simulink subsystem "lat_velocity_generator"  (R2019b)
settings: Solver=VariableStepAuto  StartTime=0.0  StopTime=10.0  RelTol=1e-3
model mask{lat_vel_error_gain=0, deadzone_bound=0, override_time=0}
  mask prompts: lat_vel_error_gain "Proportial Speed Gain"; deadzone_bound "Proportial Speed Deadzone Bound (m/s)"; override_time "Max Velocity Override Time (s)"
undefined symbols (not defined in the file): abs_yaw_params, counter_max, speed
libraries: simulink x2
settings Model: Creator=andrea  LastModifiedBy=andrea

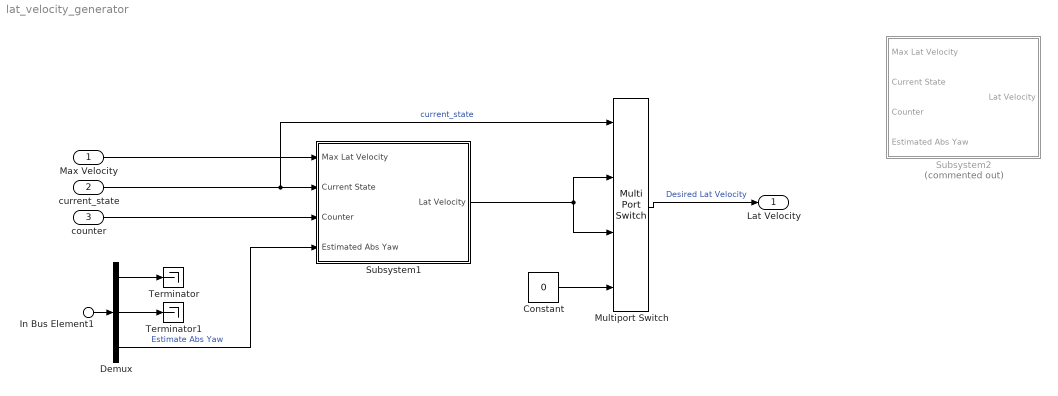
== system lat_velocity_generator ==
  Max Velocity : Inport
  current_state : Inport  Port=2
  counter : Inport  Port=3
  In Bus Element1 : Inport  Port=4  PortName=Estimates Bus  Element=Estimated Abs Orientation
  Constant : Constant  Value=0
  Demux : Demux  Outputs=3
  Multiport Switch : MultiPortSwitch  DataPortOrder=Specify indices  DataPortIndices={103, 202, 201}  DiagnosticForDefault=None
  Subsystem1 : Subsystem
  Subsystem2 : Subsystem  Commented=on
  Terminator : Terminator
  Terminator1 : Terminator
  Lat Velocity : Outport
  wires:
  Max Velocity/1 -> Subsystem1/1(Max Lat Velocity)
  current_state/1 -> Multiport Switch/1, Subsystem1/2(Current State)  "current_state"
  counter/1 -> Subsystem1/3(Counter)
  Demux/3 -> Subsystem1/4(Estimated Abs Yaw)  "Estimate Abs Yaw"
  In Bus Element1/1 -> Demux/1
  Demux/1 -> Terminator/1
  Demux/2 -> Terminator1/1
  Multiport Switch/1 -> Lat Velocity/1  "Desired Lat Velocity"
  Subsystem1/1(Lat Velocity) -> Multiport Switch/3, Multiport Switch/2
  Constant/1 -> Multiport Switch/4

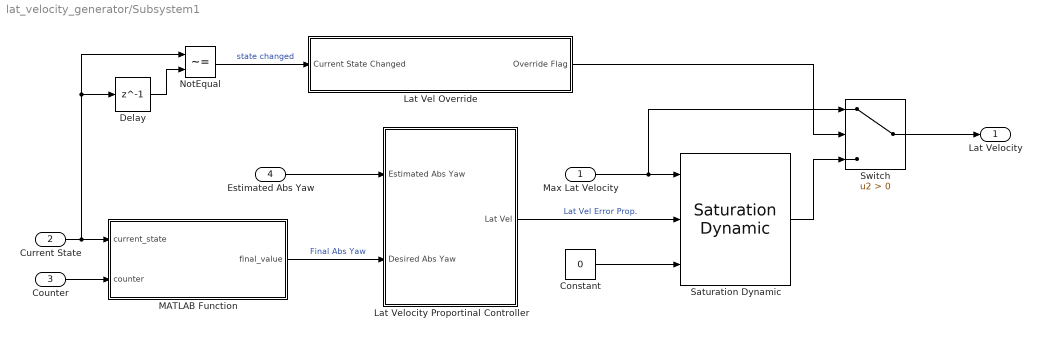
== system lat_velocity_generator/Subsystem1 ==
  Max Lat Velocity : Inport
  Current State : Inport  Port=2
  Counter : Inport  Port=3
  Estimated Abs Yaw : Inport  Port=4
  Constant : Constant  Value=0
  Delay : Delay  DelayLength=1
  Lat Vel Override : Subsystem
  Lat Velocity Proportinal Controller : Subsystem
  MATLAB Function : MATLAB Function  TreatAsAtomicUnit=on
  NotEqual : RelationalOperator  Operator=~=  OutDataTypeStr=boolean  RndMeth=Simplest
  Saturation Dynamic : simulink/Discontinuities/Saturation Dynamic  OutMin=[]  OutMax=[]  OutDataTypeStr=Inherit: Same as second input  OutDataType=fixdt(1, 16)  OutScaling=2^-10  DoSatur=off
  Switch : Switch  Criteria=u2 > Threshold
  Lat Velocity : Outport
  wires:
  Switch/1 -> Lat Velocity/1
  Lat Vel Override/1(Override Flag) -> Switch/2
  NotEqual/1 -> Lat Vel Override/1(Current State Changed)  "state changed"
  Delay/1 -> NotEqual/2
  MATLAB Function/1(final_value) -> Lat Velocity Proportinal Controller/2(Desired Abs Yaw)  "Final Abs Yaw"
  Current State/1 -> MATLAB Function/1(current_state), NotEqual/1, Delay/1
  Max Lat Velocity/1 -> Saturation Dynamic/1, Switch/1
  Saturation Dynamic/1 -> Switch/3
  Constant/1 -> Saturation Dynamic/3
  Counter/1 -> MATLAB Function/2(counter)
  Estimated Abs Yaw/1 -> Lat Velocity Proportinal Controller/1(Estimated Abs Yaw)
  Lat Velocity Proportinal Controller/1(Lat Vel) -> Saturation Dynamic/2  "Lat Vel Error Prop."

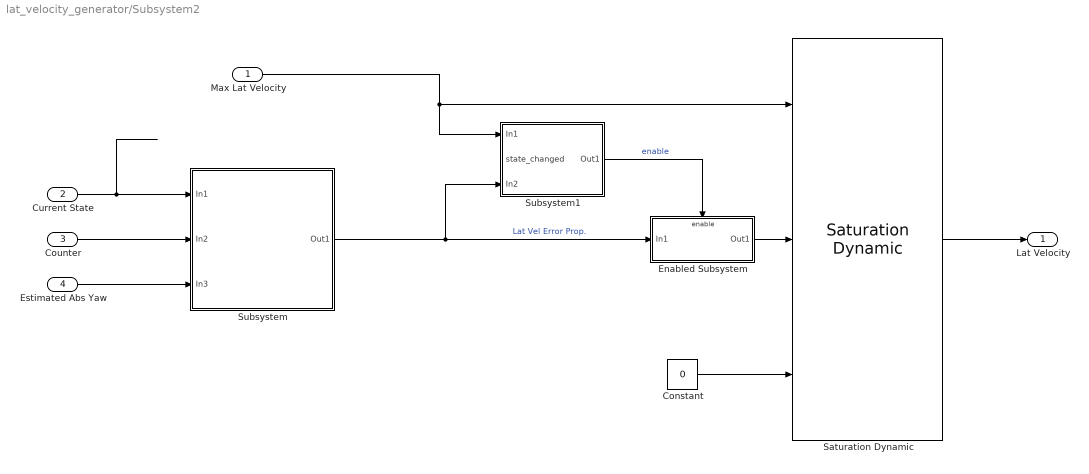
== system lat_velocity_generator/Subsystem2 ==
  Max Lat Velocity : Inport
  Current State : Inport  Port=2
  Counter : Inport  Port=3
  Estimated Abs Yaw : Inport  Port=4
  Constant : Constant  Value=0
  Enabled Subsystem : Subsystem  TreatAsAtomicUnit=on
  Saturation Dynamic : simulink/Discontinuities/Saturation Dynamic  OutMin=[]  OutMax=[]  OutDataTypeStr=Inherit: Same as second input  OutDataType=fixdt(1, 16)  OutScaling=2^-10  DoSatur=off
  Subsystem : Subsystem
  Subsystem1 : Subsystem
  Lat Velocity : Outport
  wires:
  Current State/1 -> Subsystem/1(In1)
  Max Lat Velocity/1 -> Subsystem1/1(In1), Saturation Dynamic/1
  Saturation Dynamic/1 -> Lat Velocity/1
  Constant/1 -> Saturation Dynamic/3
  Counter/1 -> Subsystem/2(In2)
  Estimated Abs Yaw/1 -> Subsystem/3(In3)
  Subsystem/1(Out1) -> Subsystem1/3(In2), Enabled Subsystem/1(In1)  "Lat Vel Error Prop."
  Enabled Subsystem/1(Out1) -> Saturation Dynamic/2
  Subsystem1/1(Out1) -> Enabled Subsystem/Enable  "enable"

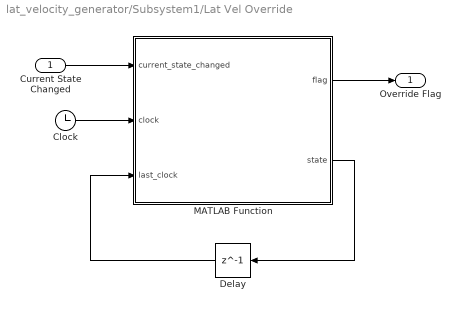
== system lat_velocity_generator/Subsystem1/Lat Vel Override ==
  Current State Changed : Inport
  Clock : Clock
  Delay : Delay  DelayLength=1
  MATLAB Function : MATLAB Function  TreatAsAtomicUnit=on
  Override Flag : Outport
  wires:
  MATLAB Function/2(state) -> Delay/1
  Delay/1 -> MATLAB Function/3(last_clock)
  Current State Changed/1 -> MATLAB Function/1(current_state_changed)
  Clock/1 -> MATLAB Function/2(clock)
  MATLAB Function/1(flag) -> Override Flag/1

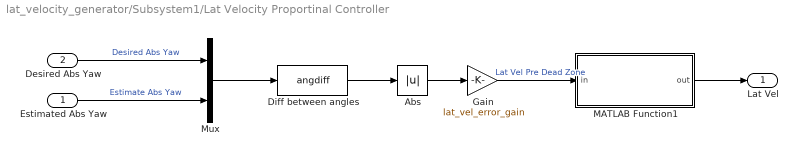
== system lat_velocity_generator/Subsystem1/Lat Velocity Proportinal Controller ==
  Estimated Abs Yaw : Inport
  Desired Abs Yaw : Inport  Port=2
  Abs : Abs
  Diff between angles : MATLABFcn  MATLABFcn=angdiff
  Gain : Gain  Gain=lat_vel_error_gain
  MATLAB Function1 : MATLAB Function  TreatAsAtomicUnit=on
  Mux : Mux  Inputs=2
  Lat Vel : Outport  OutputWhenDisabled=reset  InitialOutput=1e10
  wires:
  Desired Abs Yaw/1 -> Mux/1  "Desired Abs Yaw"
  MATLAB Function1/1(out) -> Lat Vel/1
  Diff between angles/1 -> Abs/1
  Estimated Abs Yaw/1 -> Mux/2  "Estimate Abs Yaw"
  Gain/1 -> MATLAB Function1/1(in)  "Lat Vel Pre Dead Zone"
  Abs/1 -> Gain/1
  Mux/1 -> Diff between angles/1

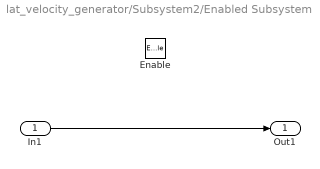
== system lat_velocity_generator/Subsystem2/Enabled Subsystem ==
  In1 : Inport
  Enable : EnablePort
  Out1 : Outport  OutputWhenDisabled=reset  InitialOutput=1e5
  wires:
  In1/1 -> Out1/1

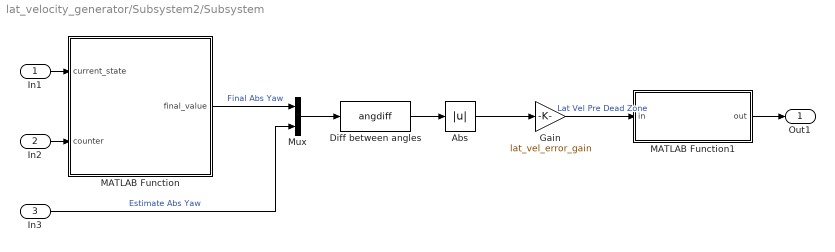
== system lat_velocity_generator/Subsystem2/Subsystem ==
  In1 : Inport
  In2 : Inport  Port=2
  In3 : Inport  Port=3
  Abs : Abs
  Diff between angles : MATLABFcn  MATLABFcn=angdiff
  Gain : Gain  Gain=lat_vel_error_gain
  MATLAB Function : MATLAB Function  TreatAsAtomicUnit=on
  MATLAB Function1 : MATLAB Function  TreatAsAtomicUnit=on
  Mux : Mux  Inputs=2
  Out1 : Outport  OutputWhenDisabled=reset  InitialOutput=1e10
  wires:
  MATLAB Function1/1(out) -> Out1/1
  Diff between angles/1 -> Abs/1
  In2/1 -> MATLAB Function/2(counter)
  In1/1 -> MATLAB Function/1(current_state)
  In3/1 -> Mux/2  "Estimate Abs Yaw"
  MATLAB Function/1(final_value) -> Mux/1  "Final Abs Yaw"
  Gain/1 -> MATLAB Function1/1(in)  "Lat Vel Pre Dead Zone"
  Abs/1 -> Gain/1
  Mux/1 -> Diff between angles/1

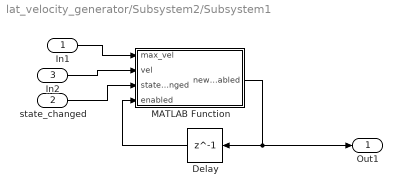
== system lat_velocity_generator/Subsystem2/Subsystem1 ==
  In1 : Inport
  state_changed : Inport  Port=2
  In2 : Inport  Port=3
  Delay : Delay  DelayLength=1  InitialCondition=0
  MATLAB Function : MATLAB Function  TreatAsAtomicUnit=on
  Out1 : Outport
  wires:
  state_changed/1 -> MATLAB Function/3(state_changed)
  Delay/1 -> MATLAB Function/4(enabled)
  In2/1 -> MATLAB Function/2(vel)
  In1/1 -> MATLAB Function/1(max_vel)
  MATLAB Function/1(new_enabled) -> Out1/1, Delay/1

== matlab function lat_velocity_generator/Subsystem1/MATLAB Function ==
  data: current_state input; counter input; abs_yaw_params parameter; counter_max parameter; final_value output
function final_value  = abs_yaw_final_value(current_state, counter, abs_yaw_params, counter_max)

row_index = checkpoint_row_index(current_state, counter, counter_max);
if row_index ~= -1
    final_value = abs_yaw_params(row_index, 2);
else
    final_value = 0;
end

end

== matlab function lat_velocity_generator/Subsystem2/Subsystem/MATLAB Function ==
  data: current_state input; counter input; abs_yaw_params parameter; counter_max parameter; final_value output
function final_value  = abs_yaw_final_value(current_state, counter, abs_yaw_params, counter_max)

row_index = checkpoint_row_index(current_state, counter, counter_max);
if row_index ~= -1
    final_value = abs_yaw_params(row_index, 2);
else
    final_value = 0;
end

end

== matlab function lat_velocity_generator/Subsystem1/Lat Velocity Proportinal Controller/MATLAB Function1 ==
  data: in input size=1; out output size=1; speed parameter; deadzone_bound parameter
function out = deadzone_with_step(in, speed, deadzone_bound)

if abs(in) < deadzone_bound
    out = 0;
else
    out = in;
end

== matlab function lat_velocity_generator/Subsystem1/Lat Vel Override/MATLAB Function ==
  data: current_state_changed input; clock input; flag output size=1; last_clock input; state output size=1; override_time parameter
function [flag, state] = fcn(current_state_changed, clock, last_clock, override_time)

if current_state_changed
    last_clock = clock + override_time;
end

state = last_clock;
if clock >= last_clock
    flag = 0;
else
    state = last_clock;
    flag = 1;
end

== matlab function lat_velocity_generator/Subsystem2/Subsystem/MATLAB Function1 ==
  data: in input size=1; out output size=1; speed parameter
function out = deadzone_with_step(in, speed)

if abs(in) < speed/2
    out = 0;
else
    out = in;
end

== matlab function lat_velocity_generator/Subsystem2/Subsystem1/MATLAB Function ==
  data: max_vel input; vel input; state_changed input; enabled input; new_enabled output
function new_enabled = fcn(max_vel, vel, state_changed, enabled)

if vel >= max_vel && enabled == 0
    new_enabled = 1;
elseif state_changed == 1
    new_enabled = 0;
else
    new_enabled = enabled;
end
